simulink model "sim_car_model2"  (R2022a)
settings: Solver=VariableStepAuto  StartTime=0.0  StopTime=500  RelTol=1e-3
values from neighbouring files (symbols this model uses):
  b = (Fmax - c*Vmax^2)/Vmax    (= 2.52478421655)    [Copy_of_script.m]    (also in script.m)
  c = 0.5*rho*A*cd    (= 0.4907934)    [Copy_of_script.m]    (also in script.m)
  g = 9.82    [Copy_of_script.m]    (also in script.m)
  m = 1001    [Copy_of_script.m]    (also in script.m)
settings Model: Creator=gomag  LastModifiedBy=gomag

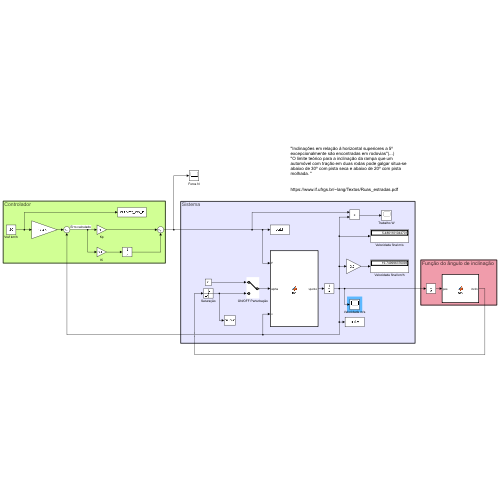
[thumbnail: Simulink's stored preview of the top-level diagram]
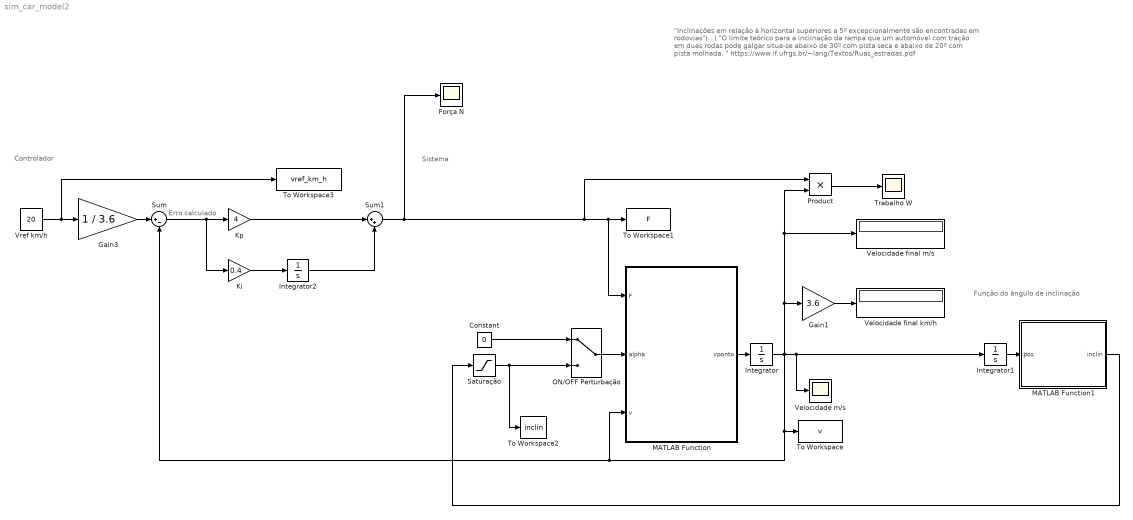
== system sim_car_model2 ==
  note: Controlador
  note: Função do ângulo de inclinação
  note: Sistema
  note: "Inclinações em relação à horizontal superiores a 5º excepcionalmente são encontradas em rodovias"(...)
      | "O limite teórico para a inclinação da rampa que um automóvel com tração em duas rodas pode galgar situa-se abaixo de 30º com pista seca e abaixo de 20º com pista molhada. "
      |
      | https://www.if.ufrgs.br/~lang/Textos/Ruas_estradas.pdf
  note: Erro calculado
  Constant : Constant  Value=0
  Força N : Scope
  Gain1 : Gain  Gain=3.6
  Gain3 : Gain  Gain=1 / 3.6
  Integrator : Integrator
  Integrator1 : Integrator
  Integrator2 : Integrator
  Ki : Gain  Gain=0.4
  Kp : Gain  Gain=4
  MATLAB Function : MATLAB Function  TreatAsAtomicUnit=on
  MATLAB Function1 : MATLAB Function  TreatAsAtomicUnit=on
  ON/OFF Perturbação : ManualSwitch
  Product : Product
  Saturação : Saturate  UpperLimit=5*pi/180  LowerLimit=-5*pi/180
  Sum : Sum  Inputs=|+-
  Sum1 : Sum  Inputs=|++
  To Workspace : ToWorkspace  VariableName=v  SaveFormat=Timeseries  SampleTime=-1
  To Workspace1 : ToWorkspace  VariableName=F  SaveFormat=Timeseries  SampleTime=-1
  To Workspace2 : ToWorkspace  VariableName=inclin  SaveFormat=Timeseries  SampleTime=-1
  To Workspace3 : ToWorkspace  VariableName=vref_km_h  SaveFormat=Timeseries  SampleTime=-1
  Trabalho W : Scope
  Velocidade final km/h : Display
      settings: Decimation=4
  Velocidade final m/s : Display
      settings: Decimation=4
  Velocidade m/s : Scope
  Vref km/h : Constant  Value=20
  wires:
  MATLAB Function/1(vponto) -> Integrator/1
  Product/1 -> Trabalho W/1
  Gain1/1 -> Velocidade final km/h/1
  Integrator1/1 -> MATLAB Function1/1(pos)
  Saturação/1 -> ON/OFF Perturbação/2, To Workspace2/1
  Integrator2/1 -> Sum1/2
  Sum1/1 -> Força N/1, MATLAB Function/1(F), To Workspace1/1, Product/1
  Sum/1 -> Kp/1, Ki/1
  Ki/1 -> Integrator2/1
  Integrator/1 -> Integrator1/1, Velocidade m/s/1, To Workspace/1, Sum/2, MATLAB Function/3(v), Gain1/1, Velocidade final m/s/1, Product/2
  Kp/1 -> Sum1/1
  Gain3/1 -> Sum/1
  MATLAB Function1/1(inclin) -> Saturação/1
  Vref km/h/1 -> To Workspace3/1, Gain3/1
  ON/OFF Perturbação/1 -> MATLAB Function/2(alpha)
  Constant/1 -> ON/OFF Perturbação/1

== matlab function sim_car_model2/MATLAB Function1 ==
  data: pos input; inclin output; freq_ang_rota parameter
function inclin = fcn(pos,freq_ang_rota)

%Atenuador de frequencia
aten=200;

%Parametros
freq= freq_ang_rota / aten;
amp= 0.1;

%Função
inclin = amp*sin(pos * freq);

== matlab function sim_car_model2/MATLAB Function ==
  data: F input; vponto output; alpha input; v input; b parameter; c parameter; m parameter; g parameter
function vponto = fcn(F, alpha, v, b, c, m, g)

vponto=( F - b*v - c*v^2 - m*g*sin(alpha) ) / m;
